simulink model "sla_vip_filter"  (R2015b)
settings: Solver=FixedStepDiscrete  StartTime=0.0  StopTime=1  RelTol=1e-3
PreLoadFcn:
  | Param_vip_pixel1
values from neighbouring files (symbols this model uses):
  Hr = fspecial('unsharp')    [Param_vip_pixel1.m]
libraries: visionsinks x5, dspsigattribs x2, dspvision x1, visionfilter x1
settings Model: Creator=amatsumo  LastModifiedBy=amatsumo
settings DataIOCC: SaveFormat=Array  SignalLoggingSaveFormat=ModelDataLogs
settings OptimizationCC: BlockReduction=off  ConditionallyExecuteInputs=off  ExpressionDepthLimit=2147483647
settings DebuggingCC: UnderspecifiedInitializationDetection=Classic  MergeDetectMultiDrivingBlocksExec=none  SolverPrmCheckMsg=warning  FcnCallInpInsideContextMsg=UseLocalSettings  StateNameClashWarn=warning
settings HardwareCC: ProdBitPerPointer=32  ProdLargestAtomicFloat=None  ProdIntDivRoundTo=Undefined  ProdEndianess=Unspecified  ProdWordSize=32  ProdHWDeviceType=ASIC/FPGA->ASIC/FPGA  TargetBitPerPointer=64  TargetLongLongMode=on  TargetIntDivRoundTo=Zero  TargetEndianess=LittleEndian  TargetWordSize=64  TargetHWDeviceType=MATLAB Host  ProdEqTarget=off
settings GRTTargetCC: GeneratePreprocessorConditionals=Disable all  CombineOutputUpdateFcns=off  GRTInterface=on
settings ConfigComp: CovModelRefEnable=Off  CovSFcnEnable=off

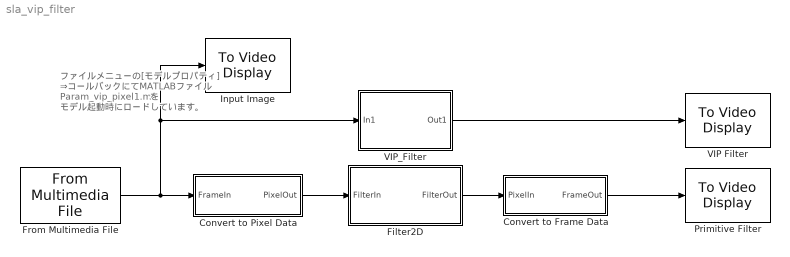
== system sla_vip_filter ==
  note: ファイルメニューの[モデルプロパティ]
      | ⇒コールバックにてMATLABファイル
      | Param_vip_pixel1.mを
      | モデル起動時にロードしています。
  Convert to Frame Data : Subsystem
  Convert to Pixel Data : Subsystem
  Filter2D : Subsystem
  From Multimedia File : dspvision/From Multimedia File  inputFilename=vipmen.avi  loop=on  numPlays=inf  outputStreams=Video only  videoDataType=uint8  audioDataType=int16  inheritSampleTime=off  userDefinedSampleTime=1/24  noAudioOutput=off  isIntensityVideo=off  fourcc=Intensity  colorVideoFormat=One multidimensional signal  outputEOF=off  dataOrg=Column-major  audioFrameSize=1024  computeAudioFrameSize=off  outSamplingMode=Frame based
  Input Image : visionsinks/To Video Display  windowSizeMode=True size (1:1)  openAtMdlStart=on  fullScreen=off  videoWindowX=367  videoWindowY=50  saveWindowSize=off  videoWindowWidth=160  videoWindowHeight=120  inputColorFormat=RGB  inputType=Obsolete  imagePorts=One multidimensional signal  OutputDevice=On-screen video monitor  dataOrg=Column-major  isWindowOpen=on
  Primitive Filter : visionsinks/To Video Display  windowSizeMode=True size (1:1)  openAtMdlStart=on  fullScreen=off  videoWindowX=1177  videoWindowY=20  saveWindowSize=off  videoWindowWidth=160  videoWindowHeight=120  inputColorFormat=RGB  inputType=Obsolete  imagePorts=One multidimensional signal  OutputDevice=On-screen video monitor  dataOrg=Column-major  isWindowOpen=on
  VIP Filter : visionsinks/To Video Display  windowSizeMode=True size (1:1)  openAtMdlStart=on  fullScreen=off  videoWindowX=642  videoWindowY=48  saveWindowSize=off  videoWindowWidth=160  videoWindowHeight=120  inputColorFormat=RGB  inputType=Obsolete  imagePorts=One multidimensional signal  OutputDevice=On-screen video monitor  dataOrg=Column-major  isWindowOpen=on
  VIP_Filter : Subsystem
  wires:
  From Multimedia File/1 -> Convert to Pixel Data/1(FrameIn), VIP_Filter/1(In1), Input Image/1
  Convert to Pixel Data/1(PixelOut) -> Filter2D/1(FilterIn)
  VIP_Filter/1(Out1) -> VIP Filter/1
  Convert to Frame Data/1(FrameOut) -> Primitive Filter/1
  Filter2D/1(FilterOut) -> Convert to Frame Data/1(PixelIn)

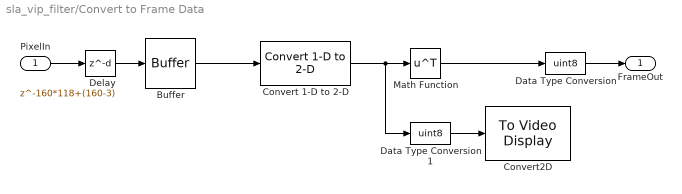
== system sla_vip_filter/Convert to Frame Data ==
  PixelIn : Inport
  Buffer : Buffer  N=160*120  TreatMby1Signals=One channel
  Convert 1-D to 2-D : dspsigattribs/Convert 1-D to 2-D  M=160  N=120  frameBasedOut=off
  Convert2D : visionsinks/To Video Display  windowSizeMode=True size (1:1)  openAtMdlStart=on  fullScreen=off  videoWindowX=807  videoWindowY=275  saveWindowSize=off  videoWindowWidth=120  videoWindowHeight=160  inputColorFormat=RGB  inputType=Obsolete  imagePorts=One multidimensional signal  OutputDevice=On-screen video monitor  dataOrg=Column-major  isWindowOpen=on
  Data Type Conversion : DataTypeConversion  OutDataTypeStr=uint8  SaturateOnIntegerOverflow=on
  Data Type Conversion1 : DataTypeConversion  OutDataTypeStr=uint8  SaturateOnIntegerOverflow=on
  Delay : Delay  DelayLength=160*118+(160-3)  InitialCondition=0
  Math Function : Math  Operator=transpose  SaturateOnIntegerOverflow=on
  FrameOut : Outport
  wires:
  Data Type Conversion/1 -> FrameOut/1
  Delay/1 -> Buffer/1
  Math Function/1 -> Data Type Conversion/1
  PixelIn/1 -> Delay/1
  Convert 1-D to 2-D/1 -> Math Function/1, Data Type Conversion1/1
  Buffer/1 -> Convert 1-D to 2-D/1
  Data Type Conversion1/1 -> Convert2D/1

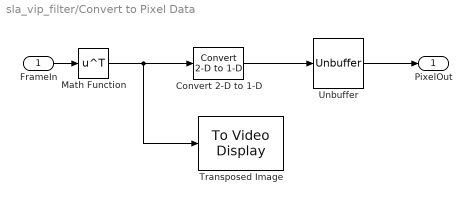
== system sla_vip_filter/Convert to Pixel Data ==
  FrameIn : Inport
  Convert 2-D to 1-D : dspsigattribs/Convert 2-D to 1-D
  Math Function : Math  Operator=transpose  SaturateOnIntegerOverflow=on
  Transposed Image : visionsinks/To Video Display  windowSizeMode=True size (1:1)  openAtMdlStart=on  fullScreen=off  videoWindowX=582  videoWindowY=275  saveWindowSize=off  videoWindowWidth=120  videoWindowHeight=160  inputColorFormat=RGB  inputType=Obsolete  imagePorts=One multidimensional signal  OutputDevice=On-screen video monitor  dataOrg=Column-major  isWindowOpen=on
  Unbuffer : Unbuffer  SampleBasedProcessing=Same as frame based
  PixelOut : Outport
  wires:
  Math Function/1 -> Convert 2-D to 1-D/1, Transposed Image/1
  Unbuffer/1 -> PixelOut/1
  FrameIn/1 -> Math Function/1
  Convert 2-D to 1-D/1 -> Unbuffer/1

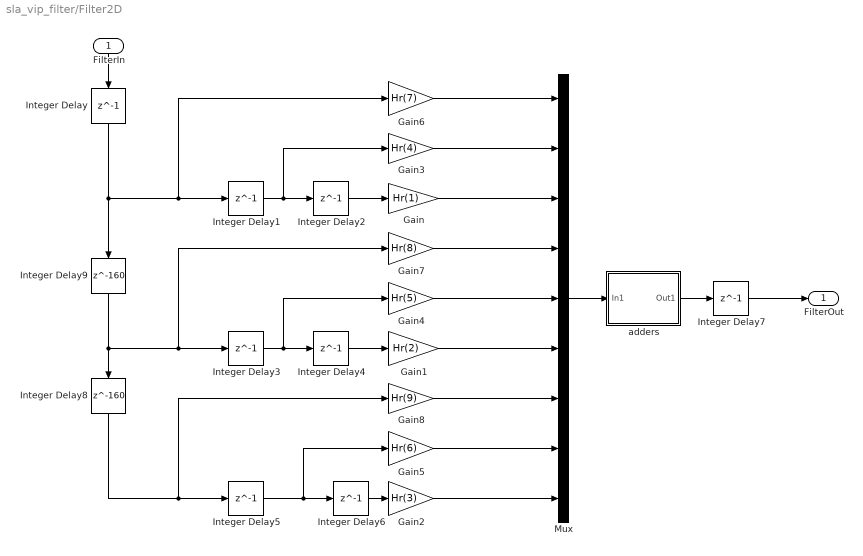
== system sla_vip_filter/Filter2D ==
  FilterIn : Inport
  Gain : Gain  Gain=Hr(1)  ParamDataTypeStr=fixdt(1,7,3)
  Gain1 : Gain  Gain=Hr(2)  ParamDataTypeStr=fixdt(1,7,3)
  Gain2 : Gain  Gain=Hr(3)  ParamDataTypeStr=fixdt(1,7,3)
  Gain3 : Gain  Gain=Hr(4)  ParamDataTypeStr=fixdt(1,7,3)  RndMeth=Nearest
  Gain4 : Gain  Gain=Hr(5)  ParamDataTypeStr=fixdt(1,7,3)
  Gain5 : Gain  Gain=Hr(6)  ParamDataTypeStr=fixdt(1,7,3)
  Gain6 : Gain  Gain=Hr(7)  ParamDataTypeStr=fixdt(1,7,3)
  Gain7 : Gain  Gain=Hr(8)  ParamDataTypeStr=fixdt(1,7,3)
  Gain8 : Gain  Gain=Hr(9)  ParamDataTypeStr=fixdt(1,7,3)
  Integer Delay{,1..7} (8 alike) : Delay  DelayLength=1  InputProcessing=Inherited
  Integer Delay8 : Delay  DelayLength=160  InputProcessing=Inherited
  Integer Delay9 : Delay  DelayLength=160  InputProcessing=Inherited
  Mux : Mux  Inputs=9
  adders : Subsystem
  FilterOut : Outport
  wires:
  Integer Delay3/1 -> Gain4/1, Integer Delay4/1
  Integer Delay5/1 -> Gain5/1, Integer Delay6/1
  Integer Delay8/1 -> Gain8/1, Integer Delay5/1
  Integer Delay9/1 -> Gain7/1, Integer Delay3/1, Integer Delay8/1
  Integer Delay1/1 -> Gain3/1, Integer Delay2/1
  FilterIn/1 -> Integer Delay/1
  Gain6/1 -> Mux/1
  Integer Delay/1 -> Gain6/1, Integer Delay1/1, Integer Delay9/1
  Integer Delay7/1 -> FilterOut/1
  Integer Delay2/1 -> Gain/1
  Gain3/1 -> Mux/2
  Gain/1 -> Mux/3
  Gain7/1 -> Mux/4
  Gain4/1 -> Mux/5
  Integer Delay4/1 -> Gain1/1
  Gain1/1 -> Mux/6
  Integer Delay6/1 -> Gain2/1
  Gain2/1 -> Mux/9
  Gain8/1 -> Mux/7
  Gain5/1 -> Mux/8
  Mux/1 -> adders/1(In1)
  adders/1(Out1) -> Integer Delay7/1

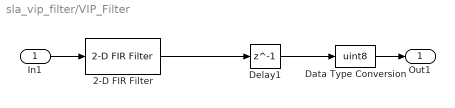
== system sla_vip_filter/VIP_Filter ==
  In1 : Inport
  2-D FIR Filter : visionfilter/2-D FIR Filter  separable=off  filtSrc=Specify via dialog  filterMtrx=Hr  verticalFilter=[4 0]  horizontalFilter=[4 0]  outSize=Same as input port I  padType=Constant  padSrc=Specify via dialog  padVal=0  method=Convolution  firstCoeffMode=Binary point scaling  firstCoeffWordLength=7  firstCoeffFracLength=3  firstCoeffSignedness=Signed  firstCoeffDataTypeStr=fixdt(1,7,3)  firstCoeffLastDataTypeStr=fixdt(1,7,3)  firstCoeffMin=[]  firstCoeffMax=[]  outputMode=Binary point scaling  outputWordLength=19  outputFracLength=8  outputSignedness=Auto  outputDataTypeStr=fixdt([],19,8)  outputLastDataTypeStr=fixdt([],19,8)  outputMin=[]  outputMax=[]  accumDataTypeStr=Inherit: Same as product output  accumLastDataTypeStr=Inherit: Same as product output  prodOutputMode=Binary point scaling  prodOutputWordLength=15  prodOutputFracLength=3  prodOutputDataTypeStr=fixdt([],15,3)  prodOutputLastDataTypeStr=fixdt([],15,3)  roundingMode=Floor  overflowMode=on
  Data Type Conversion : DataTypeConversion  OutDataTypeStr=uint8  SaturateOnIntegerOverflow=on
  Delay1 : Delay  DelayLength=1  InitialCondition=0  UseCircularBuffer=on
  Out1 : Outport
  wires:
  Delay1/1 -> Data Type Conversion/1
  2-D FIR Filter/1 -> Delay1/1
  In1/1 -> 2-D FIR Filter/1
  Data Type Conversion/1 -> Out1/1

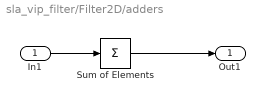
== system sla_vip_filter/Filter2D/adders ==
  In1 : Inport
  Sum of Elements : Sum  Inputs=+  RndMeth=Nearest
  Out1 : Outport
  wires:
  Sum of Elements/1 -> Out1/1
  In1/1 -> Sum of Elements/1
